simulink model "stateflowtest"  (R2018a)
settings: Solver=FixedStepDiscrete  StartTime=0.0  StopTime=10.0  FixedStep=0.1  RelTol=1e-3  EnableMultiTasking=on
settings Model: Creator=Michael Girbino  LastModifiedBy=Michael Girbino
settings SolverCC: AutoInsertRateTranBlk=on
settings DataIOCC: LimitDataPoints=on
settings OptimizationCC: LifeSpan=inf
settings DebuggingCC: AllowSymbolicDim=off  SFUnexpectedBacktrackingDiag=warning  SFNoUnconditionalDefaultTransitionDiag=warning  SFExecutionAtInitializationDiag=none
settings CodeAppCC: StateflowObjectComments=on
settings GRTTargetCC: TargetLangStandard=C89/C90 (ANSI)
settings ConfigComp: CovMetricSettings=dw  CovHtmlReporting=on  CovSaveCumulativeToWorkspaceVar=on  CovSaveSingleToWorkspaceVar=on  CovShowResultsExplorer=off  CovExternalEMLEnable=off

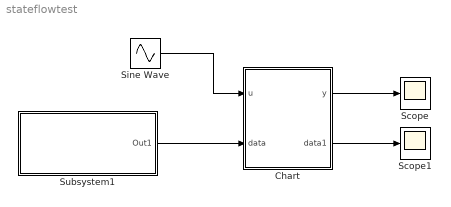
== system stateflowtest ==
  Chart : Stateflow chart  TreatAsAtomicUnit=on
  Scope : Scope
  Scope1 : Scope
  Sine Wave : Sin  SampleTime=0
  Subsystem1 : Subsystem
  wires:
  Sine Wave/1 -> Chart/1(u)
  Chart/1(y) -> Scope/1
  Chart/2(data1) -> Scope1/1
  Subsystem1/1(Out1) -> Chart/2(data)

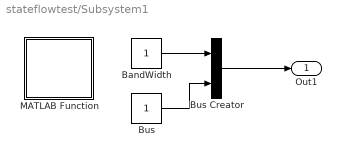
== system stateflowtest/Subsystem1 ==
  BandWidth : Constant
  Bus : Constant
  Bus Creator : BusCreator  Inputs=2  OutDataTypeStr=Bus: in2_busobj  NonVirtualBus=on
  MATLAB Function : MATLAB Function  TreatAsAtomicUnit=on
  Out1 : Outport
  wires:
  Bus Creator/1 -> Out1/1
  BandWidth/1 -> Bus Creator/1
  Bus/1 -> Bus Creator/2

== matlab function stateflowtest/Subsystem1/MATLAB Function ==
function init_params()
    band = Simulink.Parameter;
    band.DataType = double;
    set_param('stateflowtest/Bandwidth', 'Constant Value', 'band');
end

== stateflow chart stateflowtest/Chart ==
  state State1 %State Name
    entry: y = -1; % entry action
    entry: data1 = data.x;%spaghetti(data);
    % during:
  state State2
    entry: y = 1;
    entry: data1 = data.y; % 0;
  (default) -> State1 %State Name
  State1 %State Name -> State2 : [u <= 0]
      | % [transition condition]{action}
  State2 -> State1 %State Name : [u > 0]
  data: inp function_input; outp function_output; u input; y output; data input Bus: in2_busobj size=1; data1 output
  function outp = spaghetti(inp):
    | function outp = spaghetti(inp)
    |     outp = inp.x;
    | end
